simulink model "Controllo_CL_Completo_pre"  (R2024a)
settings: Solver=FixedStepAuto  StartTime=0  StopTime=30  FixedStep=1e-3  RelTol=1e-3  EnableMultiTasking=on
undefined symbols (not defined in the file): alpha_0, alpha_dot_0, cc, cm, g, L, mc, mm, xc_0, xc_dot_0
libraries: slpidlib x1, simulink x1
settings Model: Creator=Gianmarco Rallo  LastModifiedBy=smila
settings SolverCC: AlgebraicLoopSolver=TrustRegion
settings DataIOCC: LimitDataPoints=on
settings OptimizationCC: BlockReduction=off  DefaultParameterBehavior=Inlined  BufferReuse=off  LifeSpan=inf
settings DebuggingCC: UnconnectedInputMsg=warning  UnconnectedOutputMsg=warning  UnconnectedLineMsg=warning  AllowSymbolicDim=off  SFUnexpectedBacktrackingDiag=warning  SFNoUnconditionalDefaultTransitionDiag=warning  SFExecutionAtInitializationDiag=none  ArithmeticOperatorsInVariantConditions=warning
settings ModelReferenceCC: EnableRefExpFcnMdlSchedulingChecks=on  PropagateSignalLabelsOutOfModel=off
settings SFSimCC: SimUseLocalCustomCode=off  CustomCodeUndefinedFunction=UseInterfaceOnly
settings RTWCC: RTWUseLocalCustomCode=off  GPUComputeCapability=3.5
settings CodeAppCC: StateflowObjectComments=on
settings GRTTargetCC: TargetLangStandard=C89/C90 (ANSI)
settings ConfigComp: CovMetricSettings=dw  CovSaveCumulativeToWorkspaceVar=on  CovSaveSingleToWorkspaceVar=on  CovExternalEMLEnable=off

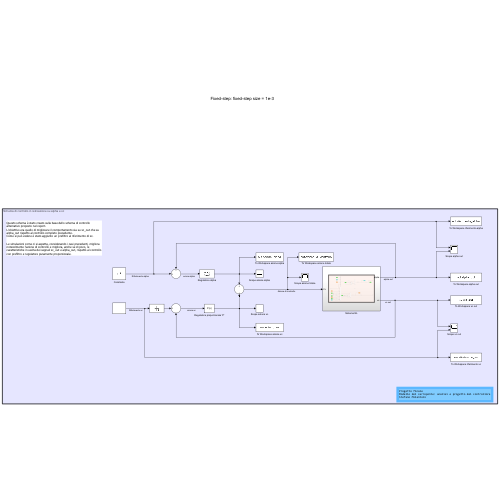
[thumbnail: Simulink's stored preview of the top-level diagram]
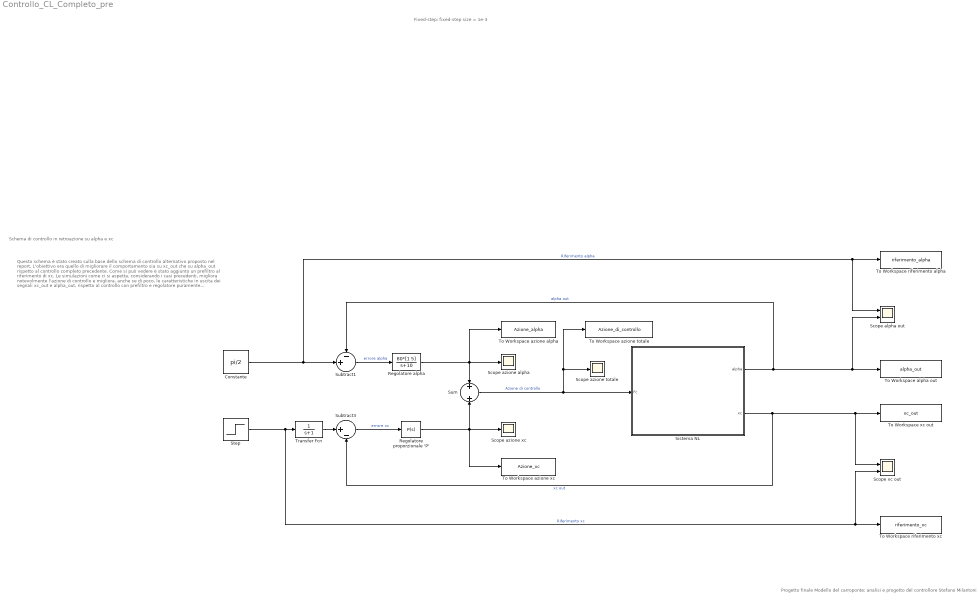
== system Controllo_CL_Completo_pre ==
  note: Questo schema è stato creato sulla base dello schema di controllo alternativo proposto nel report.
      | L'obiettivo era quello di migliorare il comportamento sia su xc_out che su alpha_out rispetto al controllo completo precedente.
      | Come si può vedere è stato aggiunto un prefiltro al riferimento di xc.
      |
      | Le simulazioni come ci si aspetta, considerando i casi precedenti, migliora notevolmente l'azione di controllo e migliora, anche se di poco, le caratteristiche in uscita dei segnali xc_out e alpha_out, rispetto al controllo con prefiltro e regolatore puramente proporzionale.
  note: Schema di controllo in retroazione su alpha e xc
  note: Fixed-step: fixed-step size = 1e-3
  note: Progetto finale
      | Modello del carroponte: analisi e progetto del controllore
      | Stefano Milantoni
  Constante : Constant  Value=pi/2
  Regolatore alpha : TransferFcn  Numerator=80*[1 5]  Denominator=[1 10]
  Regolatore proporzionale 'P' : slpidlib/PID Controller  Controller=P  Form=Parallel  TimeDomain=Continuous-time  UseExternalTs=off  SampleTime=-1  IntegratorMethod=Forward Euler  FilterMethod=Forward Euler  ControllerParametersSource=internal  P=3000  I=1  UseKiTs=off  D=0  UseExternalDerivativeSource=off  N=100  UseFilter=on  TunerSelectOption=Transfer Function Based (PID Tuner App)  InitialConditionSource=internal  InitialConditionForIntegrator=0  InitialConditionForFilter=0  DifferentiatorICPrevScaledInput=0  ExternalReset=none  TrackingMode=off  Kt=1  LimitOutput=off  SatLimitsSource=internal  UpperSaturationLimit=inf  LowerSaturationLimit=-inf  LinearizeAsGain=on  AntiWindupMode=none  Kb=1  LimitIntegrator=off  UpperIntegratorSaturationLimit=inf  LowerIntegratorSaturationLimit=-inf  POutMin=[]  POutMax=[]  IOutMin=[]  IOutMax=[]  DOutMin=[]  DOutMax=[]  NOutMin=[]  NOutMax=[]  SumOutMin=[]  SumOutMax=[]  SaturationOutMin=[]  SaturationOutMax=[]  PParamMin=[]  PParamMax=[]  IParamMin=[]  IParamMax=[]  DParamMin=[]  DParamMax=[]  NParamMin=[]  NParamMax=[]  KbParamMin=[]  KbParamMax=[]  KtParamMin=[]  KtParamMax=[]  KbOutMin=[]  KbOutMax=[]  KtOutMin=[]  KtOutMax=[]  IntegratorOutMin=[]  IntegratorOutMax=[]  FilterOutMin=[]  FilterOutMax=[]  SumI1OutMin=[]  SumI1OutMax=[]  SumI2OutMin=[]  SumI2OutMax=[]  SumI3OutMin=[]  SumI3OutMax=[]  SumI4OutMin=[]  SumI4OutMax=[]  SumDOutMin=[]  SumDOutMax=[]  DifferentiatorOutMin=[]  DifferentiatorOutMax=[]  FilterDiffOutCoefMin=[]  FilterDiffOutCoefMax=[]  ReciprocalOutMin=[]  ReciprocalOutMax=[]  SumDenOutMin=[]  SumDenOutMax=[]  SumNumOutMin=[]  SumNumOutMax=[]  DivideOutMin=[]  DivideOutMax=[]  UdiffTsProdOutMin=[]  UdiffTsProdOutMax=[]  NTsProdOutMin=[]  NTsProdOutMax=[]  UintegralTsProdOutMin=[]  UintegralTsProdOutMax=[]  UngainTsProdOutMin=[]  UngainTsProdOutMax=[]  ClampingZeroOutDataTypeStr=Inherit: Inherit via back propagation  ClampingZeroOutMin=[]  ClampingZeroOutMax=[]  FilterDenConstantOutDataTypeStr=Inherit: Inherit via back propagation  FilterDenConstantOutMin=[]  FilterDenConstantOutMax=[]  PCopyOutDataTypeStr=Inherit: Inherit via back propagation  PCopyOutMin=[]  PCopyOutMax=[]  NCopyOutDataTypeStr=Inherit: Inherit via back propagation  NCopyOutMin=[]  NCopyOutMax=[]  IntegratorContinuousStateAttributes=''  IntegratorStateMustResolveToSignalObject=off  IntegratorRTWStateStorageClass=Auto  FilterContinuousStateAttributes=''  FilterStateMustResolveToSignalObject=off  FilterRTWStateStorageClass=Auto  ParallelPVariant=InternalParameters  IdealPVariant=Disabled  IVariant=Disabled  DVariant=Disabled  IntegratorVariant=Disabled  SatVariant=Disabled  AWVariant=Disabled  PCopyVariant=Disabled  TRVariant=Disabled  FdbkBlocksVariant=Forward  IdealPFdbkVariant=Disabled  SatFdbkVariant=Disabled  DerivativeFilterVariant=Disabled  NVariant=Disabled  NCopyVariant=Disabled_SignalSpec  FilterICVariant=Disabled  IntegratorICVariant=Disabled  ExternalResetVariant=Disabled  TRSumVariant=Passthrough  SumFdbkVariant=Disabled  SumVariant=Passthrough_P  TsampFilterVariant=InternalTs  TsampNgainVariant=Passthrough  TsampIntegralVariant=Disabled_SignalSpec  ExternalSaturationOutDataTypeStr=Inherit: Same as second input  DerivativeSourceVariant=Disabled
  Scope alpha out : Scope  NumInputPorts=2
  Scope azione alpha : Scope
  Scope azione totale : Scope
  Scope azione xc : Scope
  Scope xc out : Scope  NumInputPorts=2
  Sistema NL : Subsystem
  Step : Step  Time=15  SampleTime=0
  Subtract1 : Sum  Inputs=-+|
  Subtract3 : Sum  Inputs=|+-
  Sum : Sum  Inputs=+|+
  To Workspace alpha out : ToWorkspace  VariableName=alpha_out  SaveFormat=Structure With Time  SampleTime=-1
  To Workspace azione alpha : ToWorkspace  VariableName=Azione_alpha  SaveFormat=Structure With Time  SampleTime=-1
  To Workspace azione totale : ToWorkspace  VariableName=Azione_di_controllo  SaveFormat=Structure With Time  SampleTime=-1
  To Workspace azione xc : ToWorkspace  VariableName=Azione_xc  SaveFormat=Structure With Time  SampleTime=-1
  To Workspace riferimento alpha : ToWorkspace  VariableName=riferimento_alpha  SaveFormat=Structure With Time  SampleTime=-1
  To Workspace riferimento xc : ToWorkspace  VariableName=riferimento_xc  SaveFormat=Structure With Time  SampleTime=-1
  To Workspace xc out : ToWorkspace  VariableName=xc_out  SaveFormat=Structure With Time  SampleTime=-1
  Transfer Fcn : TransferFcn  Denominator=[1 1]
  wires:
  Sistema NL/1(alpha) -> To Workspace alpha out/1, Scope alpha out/2, Subtract1/1  "alpha out"
  Sistema NL/2(xc) -> Subtract3/2, Scope xc out/1, To Workspace xc out/1  "xc out"
  Sum/1 -> Sistema NL/1(Fc), To Workspace azione totale/1, Scope azione totale/1  "Azione di controllo"
  Constante/1 -> Subtract1/2, Scope alpha out/1, To Workspace riferimento alpha/1  "Riferimento alpha"
  Step/1 -> Transfer Fcn/1, To Workspace riferimento xc/1, Scope xc out/2  "Riferimento xc"
  Subtract3/1 -> Regolatore proporzionale 'P'/1  "errore xc"
  Regolatore proporzionale 'P'/1 -> Sum/2, Scope azione xc/1, To Workspace azione xc/1
  Subtract1/1 -> Regolatore alpha/1  "errore alpha"
  Regolatore alpha/1 -> To Workspace azione alpha/1, Scope azione alpha/1, Sum/1
  Transfer Fcn/1 -> Subtract3/1

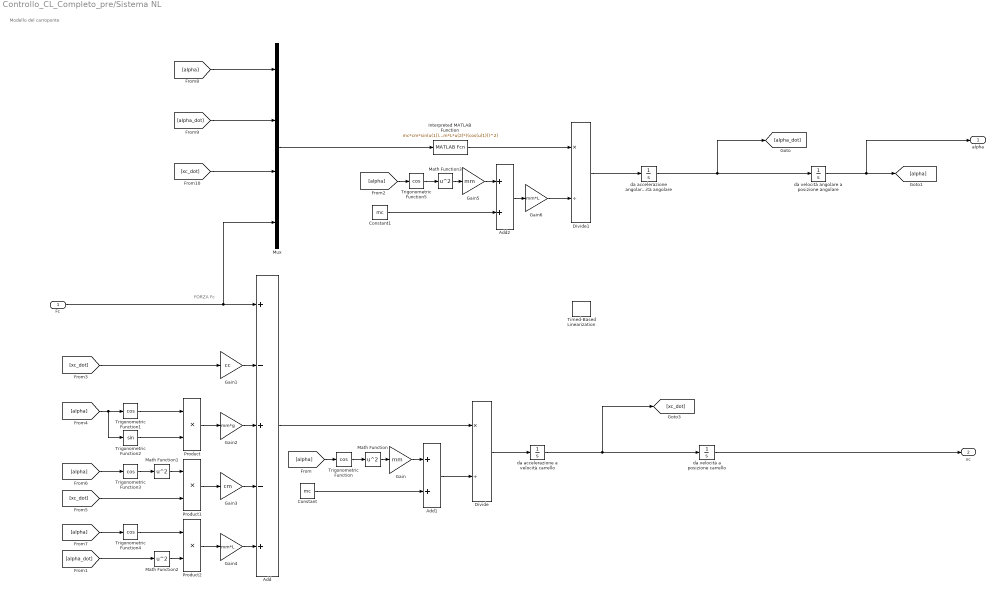
== system Controllo_CL_Completo_pre/Sistema NL ==
  note: Modello del carroponte
  note: FORZA Fc
  Fc : Inport
  Add : Sum  Inputs=+-+-+
  Add1 : Sum
  Add2 : Sum
  Constant : Constant  Value=mc
  Constant1 : Constant  Value=mc
  Divide : Product  Inputs=*/
  Divide1 : Product  Inputs=*/
  Gain : Gain  Gain=mm
  Gain1 : Gain  Gain=cc
  Gain2 : Gain  Gain=mm*g
  Gain3 : Gain  Gain=cm
  Gain4 : Gain  Gain=mm*L
  Gain5 : Gain  Gain=mm
  Gain6 : Gain  Gain=mm*L
  Interpreted MATLAB Function : MATLABFcn  MATLABFcn=mc*cm*sin(u(1))*u(3) - mm*cc*sin(u(1))*u(3) + (mm^2)*L*sin(u(1))*cos(u(1))*(u(2)^2) + mm*sin(u(1))*u(4) + (mm^2)*g*cos(u(1)) + mc*mm*g*cos(u(1)) - mc*cm*L*u(2) - mm*cm*L*u(2)*((cos(u(1)))^2)  OutputDimensions=1
  Math Function{,1..3} (4 alike) : Math  Operator=square  SignedPower=on
  Mux : Mux
  Product : Product
  Product1 : Product
  Product2 : Product
  Timed-Based Linearization : simulink/Model-Wide Utilities/Timed-Based Linearization  LinearizationTime=25  SampleTime=0
  Trigonometric Function{,1,3..5} (5 alike) : Trigonometry  Operator=cos
  Trigonometric Function2 : Trigonometry
  da accelerazione a velocità carrello : Integrator  InitialCondition=xc_dot_0
  da accelerazione angolare a velocità angolare : Integrator  InitialCondition=alpha_dot_0
  da velocità a posizione carrello : Integrator  InitialCondition=xc_0
  da velocità angolare a posizione angolare : Integrator  InitialCondition=alpha_0
  alpha : Outport
  xc : Outport  Port=2
  wires:
  Constant/1 -> Add1/2
  Math Function1/1 -> Product1/1
  Trigonometric Function2/1 -> Product/2
  Math Function/1 -> Gain/1
  [xc_dot] -> Product1/2
  Gain6/1 -> Divide1/2
  Gain1/1 -> Add/2
  Trigonometric Function5/1 -> Math Function3/1
  Math Function2/1 -> Product2/2
  [alpha] -> Trigonometric Function1/1, Trigonometric Function2/1
  Gain/1 -> Add1/1
  Trigonometric Function1/1 -> Product/1
  [alpha_dot] -> Math Function2/1
  da accelerazione a velocità carrello/1 -> [xc_dot], da velocità a posizione carrello/1
  Trigonometric Function/1 -> Math Function/1
  Divide/1 -> da accelerazione a velocità carrello/1
  Add1/1 -> Divide/2
  Product1/1 -> Gain3/1
  Fc/1 -> Add/1, Mux/4
  [alpha] -> Trigonometric Function/1
  Gain4/1 -> Add/5
  Interpreted MATLAB Function/1 -> Divide1/1
  Gain3/1 -> Add/4
  [alpha_dot] -> Mux/2
  Gain5/1 -> Add2/1
  [xc_dot] -> Mux/3
  Add/1 -> Divide/1
  [alpha] -> Trigonometric Function5/1
  da velocità angolare a posizione angolare/1 -> alpha/1, [alpha]
  Trigonometric Function3/1 -> Math Function1/1
  Math Function3/1 -> Gain5/1
  Product2/1 -> Gain4/1
  da accelerazione angolare a velocità angolare/1 -> da velocità angolare a posizione angolare/1, [alpha_dot]
  [alpha] -> Trigonometric Function4/1
  Constant1/1 -> Add2/2
  [alpha] -> Mux/1
  Gain2/1 -> Add/3
  Trigonometric Function4/1 -> Product2/1
  Product/1 -> Gain2/1
  da velocità a posizione carrello/1 -> xc/1
  [alpha] -> Trigonometric Function3/1
  [xc_dot] -> Gain1/1
  Add2/1 -> Gain6/1
  Divide1/1 -> da accelerazione angolare a velocità angolare/1
  Mux/1 -> Interpreted MATLAB Function/1
